simulink library "Collector_EN12975_r2013b"  (Simulink 8.2)
settings: Solver=ode45  StartTime=0.0  StopTime=10.0  RelTol=1e-3
libraries: carnot x4
settings Model: Creator=lena.frank  LastModifiedBy=ASIC

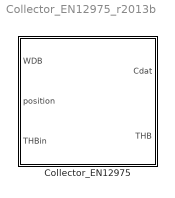
== system Collector_EN12975_r2013b ==
  Collector_EN12975 : Subsystem  mask(solar thermal collector EN 12975){acol=2.5, len=2.3, fta=0.8103, c1=3.757, c2=0.0147, c3=0, c4=0.02, c5=7062, c6=0, kblangle=[0:5:90], KbL=[1.0000    1.0000    0.9999    0.9996    0.9991    0.9982    0.9965  0.9935    0.9886    0.9807    0.9678    0.9473    0.9148    0.8638   0.7846    0.6644    0.4907    0.2599    0.0000], kbtangle=[0:5:90], KbT=[1.00000 1.00000 1.00000 1.00000 1.00000 1.00000 1.00000 1.00000 1.00000 1.00000 1.00000 0.87500 0.75000 0.62500 0.50000 0.37500 0.25000 0.12500 0], Kd=0.92, lin=0, qua=0, tini=20}
      mask prompts: acol "A : collector surface  [m²]"; len "length between inlet and outlet [m]"; fta "F'(TauAlfa)"; c1 "c1 : heat loss coefficient at (Tm-Ta)=0  [W/(m²*K)]"; c2 "c2: temperature dependence of the heat loss coefficient [W/(m*K)²]"; c3 "c3 : wind speed dependence of the heat loss coefficient [J/(m³K)]"; c4 "c4 : sky temperature dependence of the heat loss coefficient [W/(m²K)]"; c5 "c5 : effective thermal capacity [J/(m²K)]"; c6 "c6 : wind dependence of conversion factor [s/m]"; kblangle "Kb(L): angles for longitudinal IAM [degree]"; KbL "Kb(L) : incident angle modifier in longitudinal plane (beam radiation)"; kbtangle "Kb(T): angles for transversal IAM [degree]"; KbT "Kb(T) : incident angle modifier in transversal plane (beam radiation)"; Kd "Kd : Incidence angle modifier diffuse radiation"; lin "linear pressure drop in Pa/(kg/s)"; qua "quadratic pressure drop in Pa/(kg/s)²"; tini "initial temperature [degree centigrade]"
      mask help:
      | Dynamic 1-node collector model according to EN 12975 standard.
      | Energy balance:
      | mdot cp (Tout-Tin) /A = F'(TauAlfa) Kdir Idir + F'(TauAlfa) Kdfu Idfu
      |        - c1 (Tm-Tamb) - c2 (Tm-Tamb)^2 - c3 v_wind (Tm-Ta) - c6 v_wind Iglb
      |        + c4 (ELongwave - sigmaSB*(Tamb+273.15)^4) - c5 dTm/dt
      |
      | Often in test reports the optical efficiency or conversion factor eta0 is given.
      | The correlation for F'(TauAlfa) is:
      | eta0 = F'(TauAlfa) * (Kdir(15°)*0.85 + Kdfu*0.15)
      | or
      | F'(TauAlfa) = eta0 / (Kdir(15°)*0.85 + Kdfu*0.15)
      mask init:
      | acol = max(acol, 0.01);
      | c5 = max(c5, 0.001);
      mask Help: web(fullfile(path_carnot('help'),'collector_en12975.html'),'-helpbrowser')
      mask Display: disp('solar thermal\ncollector\nEN 12975\nIAM-Table')

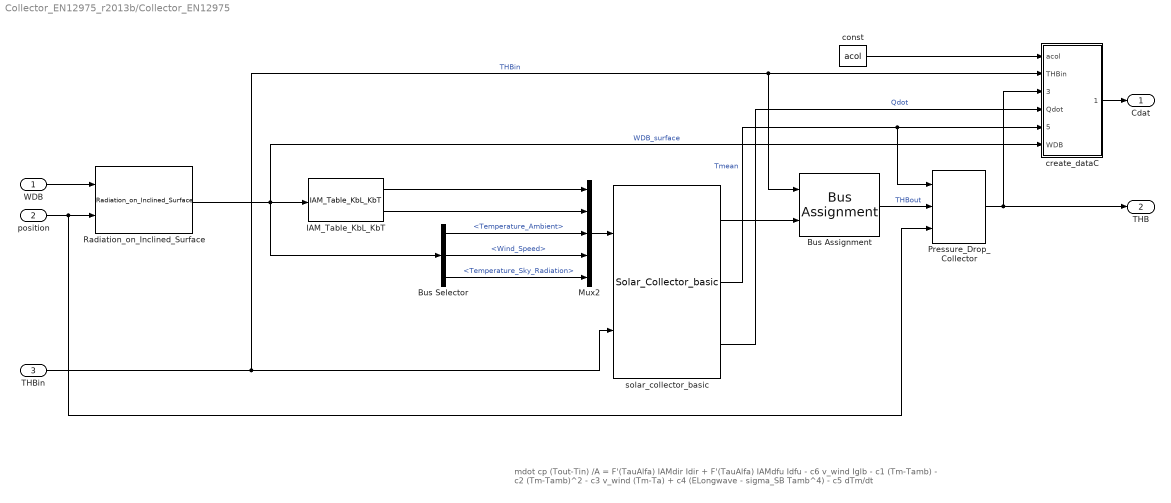
== system Collector_EN12975_r2013b/Collector_EN12975 ==
  note: mdot cp (Tout-Tin) /A = F'(TauAlfa) IAMdir Idir + F'(TauAlfa) IAMdfu Idfu - c6 v_wind Iglb - c1 (Tm-Tamb) - c2 (Tm-Tamb)^2 - c3 v_wind (Tm-Ta) + c4 (ELongwave - sigma_SB Tamb^4) - c5 dTm/dt
  WDB : Inport
  position : Inport  Port=2
  THBin : Inport  Port=3
  Bus Assignment : BusAssignment  AssignedSignals=Temperature
  Bus Selector : BusSelector  OutputSignals=Temperature_Ambient,Wind_Speed,Temperature_Sky_Radiation
  IAM_Table_KbL_KbT : carnot/Source/Solar_Thermal/IncidenceAngleModifier/IAM_Table_KbL_KbT  fta=fta  kblangle=kblangle  KbL=KbL  kbtangle=kbtangle  KbT=KbT  Kd=Kd
  Mux2 : Mux  Inputs=5
  Pressure_Drop_Collector : carnot/Basic/Pressure_Drop/Pressure_Drop_Collector  len=len  lin=lin  qua=qua
  Radiation_on_Inclined_Surface : carnot/Weather/Radiation_on_Inclined_Surface  sky=Perez 1990  reflect=0.2
  const : Constant  Value=acol
  create_dataC : Subsystem
  solar_collector_basic : carnot/Basic/Thermal_Models/Solar_Collector_basic  acol=acol  c1=c1  c2=c2  c3=c3  c4=c4  c5=c5  c6=c6  tini=tini
  Cdat : Outport  InitialOutput=0
  THB : Outport  Port=2  InitialOutput=0
  wires:
  THBin/1 -> Bus Assignment/1, create_dataC/2(THBin), solar_collector_basic/2  "THBin"
  Bus Selector/3 -> Mux2/5  "<Temperature_Sky_Radiation>"
  Bus Selector/2 -> Mux2/4  "<Wind_Speed>"
  Bus Selector/1 -> Mux2/3  "<Temperature_Ambient>"
  position/1 -> Pressure_Drop_Collector/3, Radiation_on_Inclined_Surface/2
  WDB/1 -> Radiation_on_Inclined_Surface/1
  create_dataC/1(data_c) -> Cdat/1
  IAM_Table_KbL_KbT/1 -> Mux2/1
  IAM_Table_KbL_KbT/2 -> Mux2/2
  Radiation_on_Inclined_Surface/1 -> Bus Selector/1, create_dataC/6(WDB), IAM_Table_KbL_KbT/1  "WDB_surface"
  Mux2/1 -> solar_collector_basic/1
  solar_collector_basic/3 -> create_dataC/4(Qdot)  "Qdot"
  solar_collector_basic/2 -> create_dataC/5(Tmean), Pressure_Drop_Collector/1  "Tmean"
  solar_collector_basic/1 -> Bus Assignment/2
  const/1 -> create_dataC/1(acol)
  Pressure_Drop_Collector/1 -> THB/1, create_dataC/3(THBout)
  Bus Assignment/1 -> Pressure_Drop_Collector/2  "THBout"

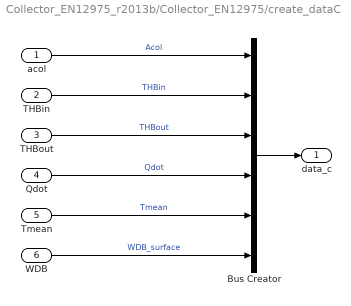
== system Collector_EN12975_r2013b/Collector_EN12975/create_dataC ==
  acol : Inport
  THBin : Inport  Port=2
  THBout : Inport  Port=3
  Qdot : Inport  Port=4
  Tmean : Inport  Port=5
  WDB : Inport  Port=6
  Bus Creator : BusCreator  Inputs=6
  data_c : Outport
  wires:
  acol/1 -> Bus Creator/1  "Acol"
  THBin/1 -> Bus Creator/2  "THBin"
  THBout/1 -> Bus Creator/3  "THBout"
  WDB/1 -> Bus Creator/6  "WDB_surface"
  Bus Creator/1 -> data_c/1
  Qdot/1 -> Bus Creator/4  "Qdot"
  Tmean/1 -> Bus Creator/5  "Tmean"
